simulink model "UAV_disturbance"  (R2018a)
settings: Solver=VariableStepAuto  StartTime=0.0  StopTime=40  RelTol=1e-3
values from neighbouring files (symbols this model uses):
  A = [0 0 1 0 0 0 0.0009 0 0 ... (first row only)    [model.m]    (also in model_disturbance.m)
  B = [0 0 0 ... (first row only)    [model.m]    (also in model_disturbance.m)
  C = [1 0 0 0 0 0 0 0 0 ... (first row only)    [model.m]    (also in model_disturbance.m)
  D = zeros(6,3)    [model.m]    (also in model_disturbance.m = zeros(6,6))
  M = A-B*K-l*C    [model.m]    (also in model_disturbance.m)
undefined symbols (not defined in the file or in its folder): K, l
settings Model: Creator=kcliu  LastModifiedBy=HP
settings CodeAppCC: StateflowObjectComments=on

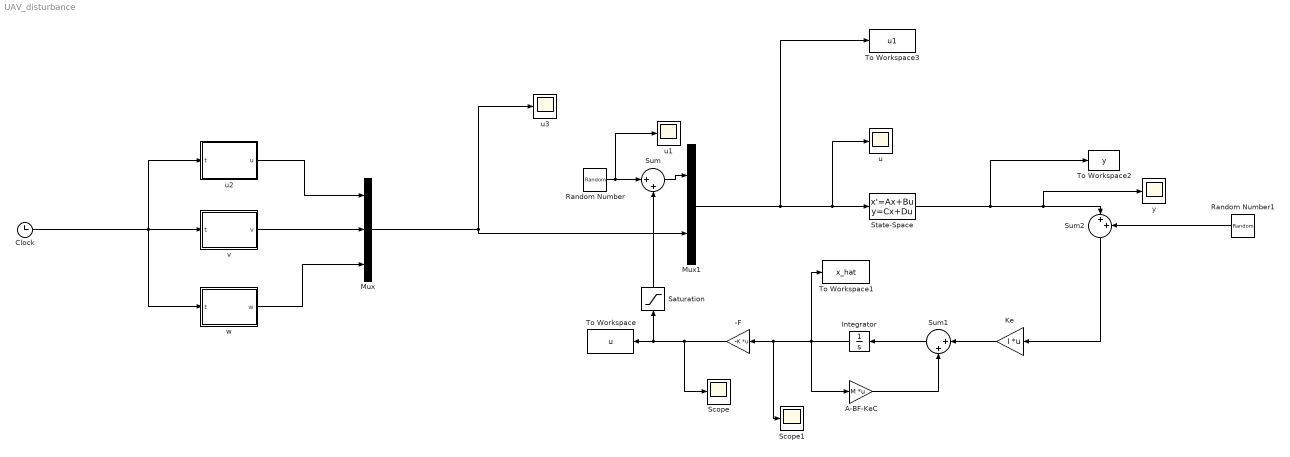
== system UAV_disturbance ==
  " -F" : Gain  Gain=-K  Multiplication=Matrix(K*u) (u vector)
  A-BF-KeC : Gain  Gain=M  Multiplication=Matrix(K*u) (u vector)
  Clock : Clock
  Integrator : Integrator  InitialCondition=[0 0 0 0 0 0 0 0 0]
  Ke : Gain  Gain=l  Multiplication=Matrix(K*u)
  Mux : Mux  Inputs=3
  Mux1 : Mux  Inputs=2
      settings: DisplayOption=signals
  Random Number : RandomNumber  Variance=0.01  SampleTime=0.1
  Random Number1 : RandomNumber  Variance=0.01  SampleTime=0.1
  Saturation : Saturate
  Scope : Scope
  Scope1 : Scope
  State-Space : StateSpace  A=A  B=[B E]  C=C  D=D  InitialCondition=[0 -0.1 0 0 0 0 0 0 0.1]  ContinuousStateAttributes='plant'
  Sum : Sum  Inputs=|++
  Sum1 : Sum  Inputs=|++
  Sum2 : Sum  Inputs=|++
  To Workspace : ToWorkspace  VariableName=u  SampleTime=-1
  To Workspace1 : ToWorkspace  VariableName=x_hat  SampleTime=-1
  To Workspace2 : ToWorkspace  VariableName=y  SampleTime=-1
  To Workspace3 : ToWorkspace  VariableName=u1  SampleTime=-1
  u : Scope
  u1 : Scope
  u2 : MATLAB Function  TreatAsAtomicUnit=on
  u3 : Scope
  v : MATLAB Function  TreatAsAtomicUnit=on
  w : MATLAB Function  TreatAsAtomicUnit=on
  y : Scope
  wires:
  Random Number/1 -> u1/1, Sum/1
  State-Space/1 -> To Workspace2/1, y/1, Sum2/1
  Random Number1/1 -> Sum2/2
  Sum2/1 -> Ke/1
  Ke/1 -> Sum1/1
  A-BF-KeC/1 -> Sum1/2
  Sum1/1 -> Integrator/1
  Integrator/1 -> Scope1/1, " -F"/1, A-BF-KeC/1, To Workspace1/1
  " -F"/1 -> Scope/1, To Workspace/1, Saturation/1
  Saturation/1 -> Sum/2
  w/1(w) -> Mux/3
  u2/1(u) -> Mux/1
  v/1(v) -> Mux/2
  Clock/1 -> w/1(t), u2/1(t), v/1(t)
  Mux1/1 -> u/1, State-Space/1, To Workspace3/1
  Sum/1 -> Mux1/1
  Mux/1 -> u3/1, Mux1/2

== matlab function UAV_disturbance/v ==
  data: t input; v output
function v = fcn(t)
if (t>=10&&t<=30)
v =10*cos(2*pi/40*(t-20));
else
    v=0;
end

== matlab function UAV_disturbance/u2 ==
  data: t input; u output
function u = fcn(t)
if (t>=10&&t<=30)
u =10*cos(2*pi/40*(t-20));
else
    u=0;
end

== matlab function UAV_disturbance/w ==
  data: t input; w output
function w = fcn(t)
if (t>=10&&t<=30)
w = 3*cos(2*pi/40*(t-20));
else
    w=0;
end
